simulink model "robusni_of_SMC_regulacija_nelin_sim"  (R2020a)
settings: Solver=ode5  StartTime=0.0  StopTime=tfin  FixedStep=1e-4  RelTol=1e-3
values from neighbouring files (symbols this model uses):
  beta = S_upper_limit*w0/2    (= 0.065530125)    [SMC_regulacija_nelin_sim_matlab.m]    (also in robusni_of_SMC_regulacija_nelin_sim_matlab.m)
  disturb_X = 0.2*Xe    (= 0.97814)    [SMC_regulacija_nelin_sim_matlab.m]    (also in robusni_of_SMC_regulacija_nelin_sim_matlab.m)
  F_lower_limit = 0    [SMC_regulacija_nelin_sim_matlab.m]    (also in robusni_of_SMC_regulacija_nelin_sim_matlab.m)
  F_upper_limit = Fe+1e-3*Fe    (= 3.2121089)    [SMC_regulacija_nelin_sim_matlab.m]    (also in robusni_of_SMC_regulacija_nelin_sim_matlab.m)
  Fi = beta/5/w0    (= 0.02325)    [SMC_regulacija_nelin_sim_matlab.m]    (also in robusni_of_SMC_regulacija_nelin_sim_matlab.m)
  K1 = 0.03    [SMC_regulacija_nelin_sim_matlab.m]    (also in robusni_of_SMC_regulacija_nelin_sim_matlab.m)
  K2 = 0.5    [SMC_regulacija_nelin_sim_matlab.m]    (also in robusni_of_SMC_regulacija_nelin_sim_matlab.m)
  mi_max = 1    [SMC_regulacija_nelin_sim_matlab.m]    (also in robusni_of_SMC_regulacija_nelin_sim_matlab.m)
  S_step = 0    [SMC_regulacija_nelin_sim_matlab.m]    (also in robusni_of_SMC_regulacija_nelin_sim_matlab.m)
  S_time_step1 = 2    [SMC_regulacija_nelin_sim_matlab.m]    (also in robusni_of_SMC_regulacija_nelin_sim_matlab.m = 20)
  S_time_step2 = 40    [SMC_regulacija_nelin_sim_matlab.m]    (also in robusni_of_SMC_regulacija_nelin_sim_matlab.m = 50)
  Se = 0.2187    [SMC_regulacija_nelin_sim_matlab.m]    (also in robusni_of_SMC_regulacija_nelin_sim_matlab.m)
  SF = 10    [SMC_regulacija_nelin_sim_matlab.m]    (also in robusni_of_SMC_regulacija_nelin_sim_matlab.m)
  std_noise = 0    [SMC_regulacija_nelin_sim_matlab.m]    (also in robusni_of_SMC_regulacija_nelin_sim_matlab.m)
  V = 4    [SMC_regulacija_nelin_sim_matlab.m]    (also in robusni_of_SMC_regulacija_nelin_sim_matlab.m)
  x10 = Xe    (= 4.8907)    [SMC_regulacija_nelin_sim_matlab.m]    (also in robusni_of_SMC_regulacija_nelin_sim_matlab.m)
  x20 = Se    (= 0.2187)    [SMC_regulacija_nelin_sim_matlab.m]    (also in robusni_of_SMC_regulacija_nelin_sim_matlab.m)
  Y = 0.5    [SMC_regulacija_nelin_sim_matlab.m]    (also in robusni_of_SMC_regulacija_nelin_sim_matlab.m)
  Y1 = Y - 0.2*Y    (= 0.4)    [robusni_of_SMC_regulacija_nelin_sim_matlab.m]
  Y2 = Y - 0.1*Y    (= 0.45)    [robusni_of_SMC_regulacija_nelin_sim_matlab.m]
  Y3 = Y + 0.1*Y    (= 0.55)    [robusni_of_SMC_regulacija_nelin_sim_matlab.m]
  Y4 = Y + 0.2*Y    (= 0.6)    [robusni_of_SMC_regulacija_nelin_sim_matlab.m]
undefined symbols (not defined in the file or in its folder): magnitude
settings Model: Creator=anaMceranic  LastModifiedBy=anaMceranic
settings DataIOCC: ReturnWorkspaceOutputs=off

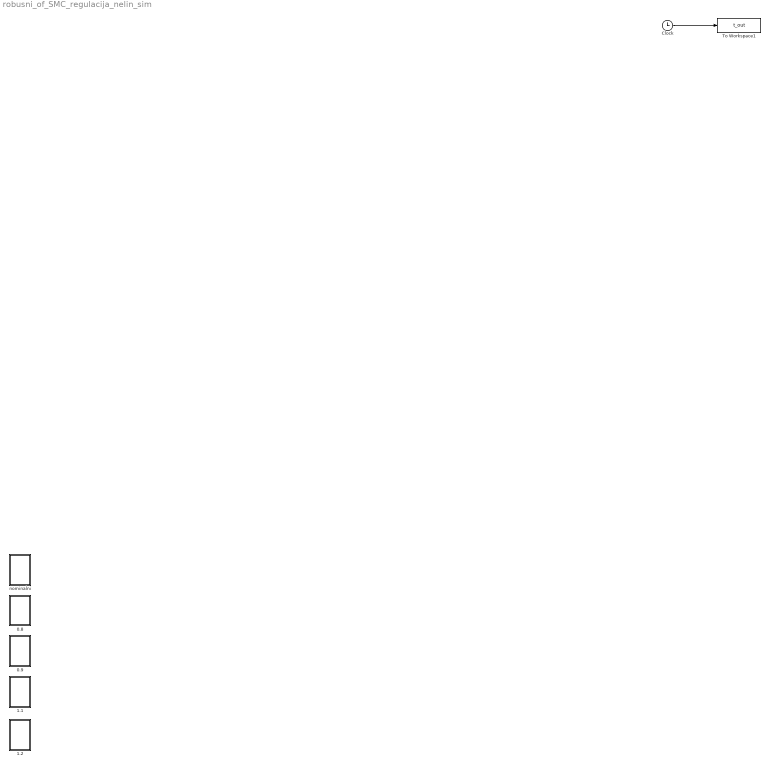
== system robusni_of_SMC_regulacija_nelin_sim ==
  0.8 : Subsystem
  0.9 : Subsystem
  1.1 : Subsystem
  1.2 : Subsystem
  Clock : Clock
  To Workspace1 : ToWorkspace  VariableName=t_out  SampleTime=-1
  nominalni : Subsystem
  wires:
  Clock/1 -> To Workspace1/1

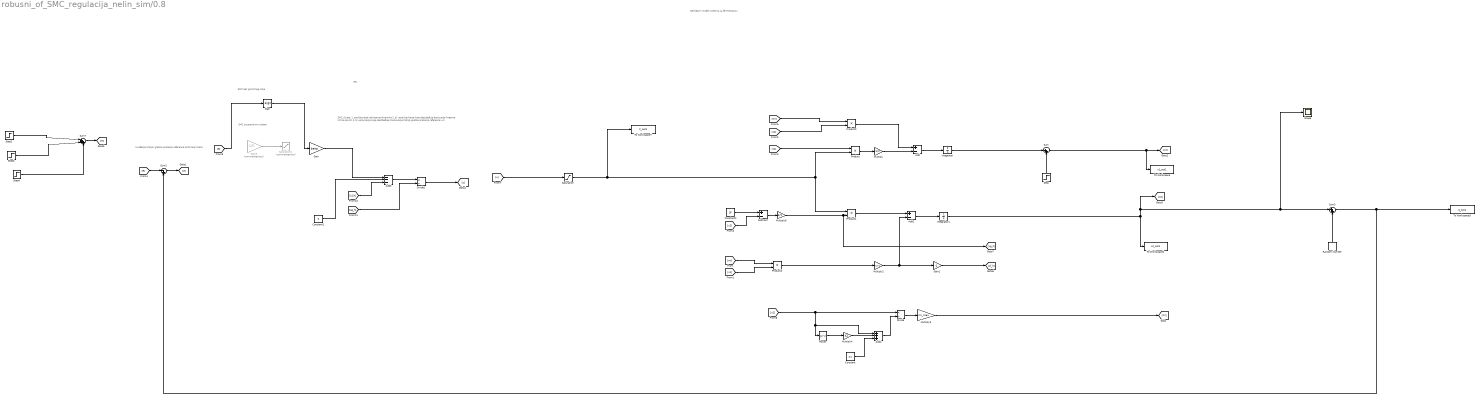
== system robusni_of_SMC_regulacija_nelin_sim/0.8 ==
  note: Nelinearni model sistema za fermentaciju
  note: SMC skupa:
      | 1. poništavanje nelinearne dinamike
      | 2. a) upravljavljanje koje obezbeđuje dostizanje linearne klizne površi
      | 2. b) upravljanje koje obezbeđuje zavšavanje stanja greške praćenja reference u 0
  note: eFL
  note: SMC bez graničnog sloja
  note: SMC sa graničnim slojem
  note: Uvođenje stanja:
      | greška praćenja reference od strane izlaza
  Add : Sum  Inputs=+-
  Add1 : Sum  Inputs=+-
  Add2 : Sum  Inputs=+++
  Add3 : Sum  Inputs=---
  Constant : Constant  Value=K1
  Constant1 : Constant  Value=0
  Constant2 : Constant  Value=SF
  Divide : Product  Inputs=*/
  Divide1 : Product  Inputs=*/
  Gain : Gain  Gain=beta
  Gain1 : Gain  Gain=-1
  Gain3 : Gain  Commented=on  Gain=1/Fi
  Integrator : Integrator  InitialCondition=x10
  Integrator1 : Integrator  InitialCondition=x20
  Multiply : Gain  Gain=1/V
  Multiply2 : Gain  Gain=1/Y1
  Multiply3 : Gain  Gain=mi_max
  Multiply4 : Gain  Gain=K2
  Multiply6 : Gain  Gain=1/V
  Power : Math  Operator=magnitude^2  SaturateOnIntegerOverflow=on
  Product{,1..3} (4 alike) : Product
  Random Number : RandomNumber  Variance=std_noise  SampleTime=0.1
  Saturation : Saturate  UpperLimit=F_upper_limit  LowerLimit=F_lower_limit
  Saturation1 : Saturate  Commented=on
  Scope : Scope
  Sign : Signum
  Step : Step  Time=5  After=disturb_X  SampleTime=0
  Step2 : Step  Time=0  Before=Se  After=Se  SampleTime=0
  Step3 : Step  Time=S_time_step1  After=S_step  SampleTime=0
  Step4 : Step  Time=S_time_step2  After=-S_step  SampleTime=0
  Subtract : Sum  Inputs=+-
  Sum : Sum  Inputs=|++
  Sum2 : Sum  Inputs=|-+
  Sum3 : Sum  Inputs=|++
  Sum7 : Sum  Inputs=|+++
  To Workspace : ToWorkspace  VariableName=x1_out1  SampleTime=-1
  To Workspace2 : ToWorkspace  VariableName=x2_out1  SampleTime=-1
  To Workspace3 : ToWorkspace  VariableName=S_out1  SampleTime=-1
  To Workspace7 : ToWorkspace  VariableName=F_out1  SampleTime=-1
  wires:
  [u] -> Saturation/1
  Random Number/1 -> Sum3/2
  [mi] -> Product3/1
  Product/1 -> Multiply/1
  Add3/1 -> Divide1/1
  Sum2/1 -> [e]
  Divide/1 -> Multiply3/1
  Add/1 -> Integrator/1
  Divide1/1 -> [u]
  Add1/1 -> Integrator1/1
  Product1/1 -> Add1/1
  Integrator/1 -> Sum/1
  Multiply4/1 -> Add2/2
  Constant2/1 -> Subtract/1
  Multiply6/1 -> Product1/2, [Lg_h]
  Constant/1 -> Add2/3
  [x1] -> Product/1
  Step/1 -> Sum/2
  [x2] -> Divide/1, Add2/1, Power/1
  [Lf_h] -> Add3/3
  [x2] -> Subtract/2
  Product2/1 -> Multiply2/1
  Add2/1 -> Divide/2
  Gain3/1 -> Saturation1/1
  Sum/1 -> To Workspace/1, [x1]
  [x1] -> Product3/2
  Sum3/1 -> To Workspace3/1, Sum2/2
  Step4/1 -> Sum7/3
  Integrator1/1 -> To Workspace2/1, [x2], Sum3/1, Scope/1
  Multiply3/1 -> [mi]
  [x1] -> Product2/2
  [Lg_h] -> Divide1/2
  Multiply2/1 -> Add1/2, Gain1/1
  Step3/1 -> Sum7/2
  Gain/1 -> Add3/1
  Product3/1 -> Add/1
  [R] -> Sum2/1
  Subtract/1 -> Multiply6/1
  Multiply/1 -> Add/2
  Saturation/1 -> Product/2, Product1/1, To Workspace7/1
  Gain1/1 -> [Lf_h]
  Sum7/1 -> [R]
  Constant1/1 -> Add3/2
  Step2/1 -> Sum7/1
  [mi] -> Product2/1
  Power/1 -> Multiply4/1
  [e] -> Sign/1
  Sign/1 -> Gain/1

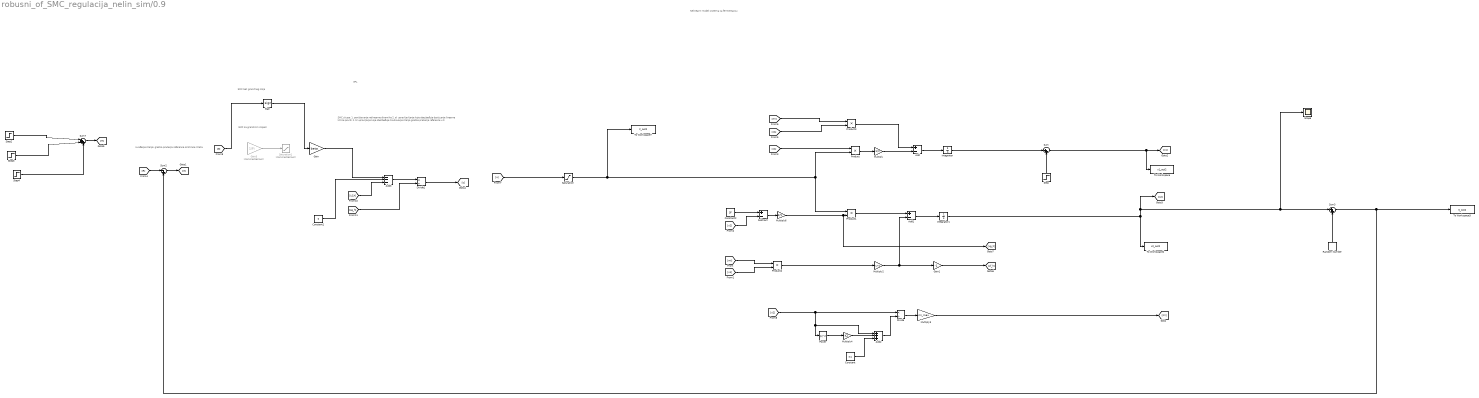
== system robusni_of_SMC_regulacija_nelin_sim/0.9 ==
  note: Uvođenje stanja:
      | greška praćenja reference od strane izlaza
  note: SMC sa graničnim slojem
  note: SMC bez graničnog sloja
  note: eFL
  note: SMC skupa:
      | 1. poništavanje nelinearne dinamike
      | 2. a) upravljavljanje koje obezbeđuje dostizanje linearne klizne površi
      | 2. b) upravljanje koje obezbeđuje zavšavanje stanja greške praćenja reference u 0
  note: Nelinearni model sistema za fermentaciju
  Add : Sum  Inputs=+-
  Add1 : Sum  Inputs=+-
  Add2 : Sum  Inputs=+++
  Add3 : Sum  Inputs=---
  Constant : Constant  Value=K1
  Constant1 : Constant  Value=0
  Constant2 : Constant  Value=SF
  Divide : Product  Inputs=*/
  Divide1 : Product  Inputs=*/
  Gain : Gain  Gain=beta
  Gain1 : Gain  Gain=-1
  Gain3 : Gain  Commented=on  Gain=1/Fi
  Integrator : Integrator  InitialCondition=x10
  Integrator1 : Integrator  InitialCondition=x20
  Multiply : Gain  Gain=1/V
  Multiply2 : Gain  Gain=1/Y2
  Multiply3 : Gain  Gain=mi_max
  Multiply4 : Gain  Gain=K2
  Multiply6 : Gain  Gain=1/V
  Power : Math  Operator=magnitude^2  SaturateOnIntegerOverflow=on
  Product{,1..3} (4 alike) : Product
  Random Number : RandomNumber  Variance=std_noise  SampleTime=0.1
  Saturation : Saturate  UpperLimit=F_upper_limit  LowerLimit=F_lower_limit
  Saturation1 : Saturate  Commented=on
  Scope : Scope
  Sign : Signum
  Step : Step  Time=5  After=disturb_X  SampleTime=0
  Step2 : Step  Time=0  Before=Se  After=Se  SampleTime=0
  Step3 : Step  Time=S_time_step1  After=S_step  SampleTime=0
  Step4 : Step  Time=S_time_step2  After=-S_step  SampleTime=0
  Subtract : Sum  Inputs=+-
  Sum : Sum  Inputs=|++
  Sum2 : Sum  Inputs=|-+
  Sum3 : Sum  Inputs=|++
  Sum7 : Sum  Inputs=|+++
  To Workspace : ToWorkspace  VariableName=x1_out2  SampleTime=-1
  To Workspace2 : ToWorkspace  VariableName=x2_out2  SampleTime=-1
  To Workspace3 : ToWorkspace  VariableName=S_out2  SampleTime=-1
  To Workspace7 : ToWorkspace  VariableName=F_out2  SampleTime=-1
  wires:
  Power/1 -> Multiply4/1
  [mi] -> Product2/1
  Step2/1 -> Sum7/1
  Constant1/1 -> Add3/2
  Sum7/1 -> [R]
  Gain1/1 -> [Lf_h]
  Saturation/1 -> To Workspace7/1, Product1/1, Product/2
  Multiply/1 -> Add/2
  Subtract/1 -> Multiply6/1
  [R] -> Sum2/1
  Product3/1 -> Add/1
  Gain/1 -> Add3/1
  Step3/1 -> Sum7/2
  Multiply2/1 -> Gain1/1, Add1/2
  [Lg_h] -> Divide1/2
  [x1] -> Product2/2
  Multiply3/1 -> [mi]
  Integrator1/1 -> Scope/1, Sum3/1, [x2], To Workspace2/1
  Step4/1 -> Sum7/3
  Sum3/1 -> Sum2/2, To Workspace3/1
  [x1] -> Product3/2
  Sum/1 -> [x1], To Workspace/1
  Gain3/1 -> Saturation1/1
  Add2/1 -> Divide/2
  Product2/1 -> Multiply2/1
  [x2] -> Subtract/2
  [Lf_h] -> Add3/3
  [x2] -> Power/1, Add2/1, Divide/1
  Step/1 -> Sum/2
  [x1] -> Product/1
  Constant/1 -> Add2/3
  Multiply6/1 -> [Lg_h], Product1/2
  Constant2/1 -> Subtract/1
  Multiply4/1 -> Add2/2
  Integrator/1 -> Sum/1
  Product1/1 -> Add1/1
  Add1/1 -> Integrator1/1
  Divide1/1 -> [u]
  Add/1 -> Integrator/1
  Divide/1 -> Multiply3/1
  Sum2/1 -> [e]
  Add3/1 -> Divide1/1
  Product/1 -> Multiply/1
  [mi] -> Product3/1
  Random Number/1 -> Sum3/2
  [u] -> Saturation/1
  [e] -> Sign/1
  Sign/1 -> Gain/1

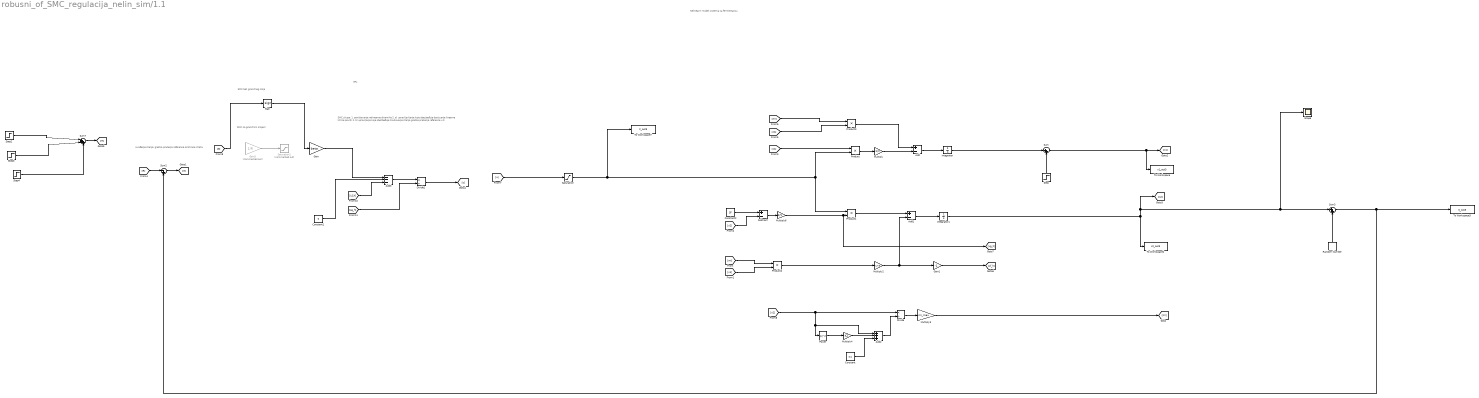
== system robusni_of_SMC_regulacija_nelin_sim/1.1 ==
  note: Nelinearni model sistema za fermentaciju
  note: SMC skupa:
      | 1. poništavanje nelinearne dinamike
      | 2. a) upravljavljanje koje obezbeđuje dostizanje linearne klizne površi
      | 2. b) upravljanje koje obezbeđuje zavšavanje stanja greške praćenja reference u 0
  note: eFL
  note: SMC bez graničnog sloja
  note: SMC sa graničnim slojem
  note: Uvođenje stanja:
      | greška praćenja reference od strane izlaza
  Add : Sum  Inputs=+-
  Add1 : Sum  Inputs=+-
  Add2 : Sum  Inputs=+++
  Add3 : Sum  Inputs=---
  Constant : Constant  Value=K1
  Constant1 : Constant  Value=0
  Constant2 : Constant  Value=SF
  Divide : Product  Inputs=*/
  Divide1 : Product  Inputs=*/
  Gain : Gain  Gain=beta
  Gain1 : Gain  Gain=-1
  Gain3 : Gain  Commented=on  Gain=1/Fi
  Integrator : Integrator  InitialCondition=x10
  Integrator1 : Integrator  InitialCondition=x20
  Multiply : Gain  Gain=1/V
  Multiply2 : Gain  Gain=1/Y3
  Multiply3 : Gain  Gain=mi_max
  Multiply4 : Gain  Gain=K2
  Multiply6 : Gain  Gain=1/V
  Power : Math  Operator=magnitude^2  SaturateOnIntegerOverflow=on
  Product{,1..3} (4 alike) : Product
  Random Number : RandomNumber  Variance=std_noise  SampleTime=0.1
  Saturation : Saturate  UpperLimit=F_upper_limit  LowerLimit=F_lower_limit
  Saturation1 : Saturate  Commented=on
  Scope : Scope
  Sign : Signum
  Step : Step  Time=5  After=disturb_X  SampleTime=0
  Step2 : Step  Time=0  Before=Se  After=Se  SampleTime=0
  Step3 : Step  Time=S_time_step1  After=S_step  SampleTime=0
  Step4 : Step  Time=S_time_step2  After=-S_step  SampleTime=0
  Subtract : Sum  Inputs=+-
  Sum : Sum  Inputs=|++
  Sum2 : Sum  Inputs=|-+
  Sum3 : Sum  Inputs=|++
  Sum7 : Sum  Inputs=|+++
  To Workspace : ToWorkspace  VariableName=x1_out3  SampleTime=-1
  To Workspace2 : ToWorkspace  VariableName=x2_out3  SampleTime=-1
  To Workspace3 : ToWorkspace  VariableName=S_out3  SampleTime=-1
  To Workspace7 : ToWorkspace  VariableName=F_out3  SampleTime=-1
  wires:
  [u] -> Saturation/1
  Random Number/1 -> Sum3/2
  [mi] -> Product3/1
  Product/1 -> Multiply/1
  Add3/1 -> Divide1/1
  Sum2/1 -> [e]
  Divide/1 -> Multiply3/1
  Add/1 -> Integrator/1
  Divide1/1 -> [u]
  Add1/1 -> Integrator1/1
  Product1/1 -> Add1/1
  Integrator/1 -> Sum/1
  Multiply4/1 -> Add2/2
  Constant2/1 -> Subtract/1
  Multiply6/1 -> Product1/2, [Lg_h]
  Constant/1 -> Add2/3
  [x1] -> Product/1
  Step/1 -> Sum/2
  [x2] -> Divide/1, Add2/1, Power/1
  [Lf_h] -> Add3/3
  [x2] -> Subtract/2
  Product2/1 -> Multiply2/1
  Add2/1 -> Divide/2
  Gain3/1 -> Saturation1/1
  Sum/1 -> To Workspace/1, [x1]
  [x1] -> Product3/2
  Sum3/1 -> To Workspace3/1, Sum2/2
  Step4/1 -> Sum7/3
  Integrator1/1 -> To Workspace2/1, [x2], Sum3/1, Scope/1
  Multiply3/1 -> [mi]
  [x1] -> Product2/2
  [Lg_h] -> Divide1/2
  Multiply2/1 -> Add1/2, Gain1/1
  Step3/1 -> Sum7/2
  Gain/1 -> Add3/1
  Product3/1 -> Add/1
  [R] -> Sum2/1
  Subtract/1 -> Multiply6/1
  Multiply/1 -> Add/2
  Saturation/1 -> Product/2, Product1/1, To Workspace7/1
  Gain1/1 -> [Lf_h]
  Sum7/1 -> [R]
  Constant1/1 -> Add3/2
  Step2/1 -> Sum7/1
  [mi] -> Product2/1
  Power/1 -> Multiply4/1
  [e] -> Sign/1
  Sign/1 -> Gain/1

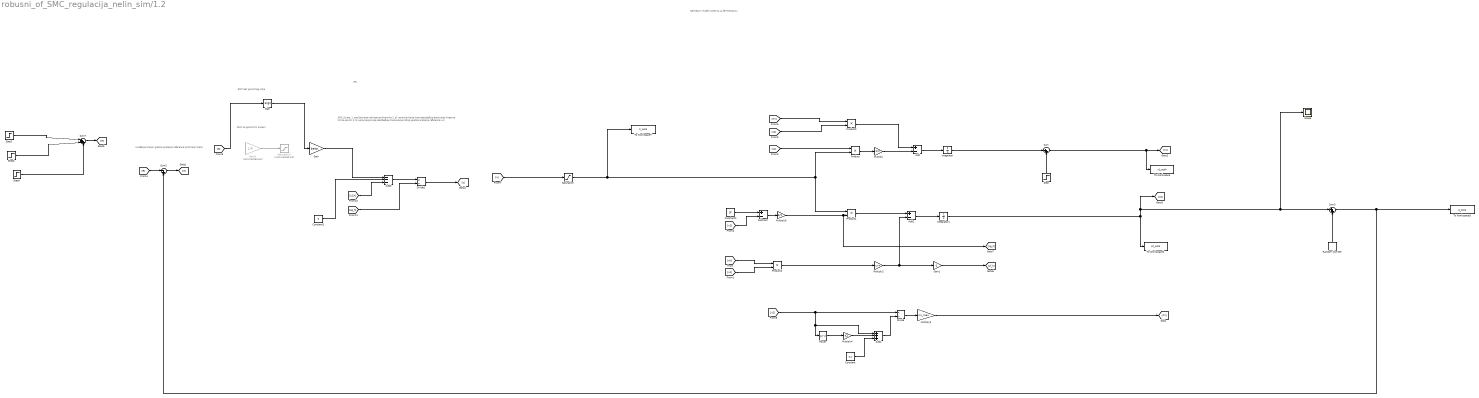
== system robusni_of_SMC_regulacija_nelin_sim/1.2 ==
  note: Uvođenje stanja:
      | greška praćenja reference od strane izlaza
  note: SMC sa graničnim slojem
  note: SMC bez graničnog sloja
  note: eFL
  note: SMC skupa:
      | 1. poništavanje nelinearne dinamike
      | 2. a) upravljavljanje koje obezbeđuje dostizanje linearne klizne površi
      | 2. b) upravljanje koje obezbeđuje zavšavanje stanja greške praćenja reference u 0
  note: Nelinearni model sistema za fermentaciju
  Add : Sum  Inputs=+-
  Add1 : Sum  Inputs=+-
  Add2 : Sum  Inputs=+++
  Add3 : Sum  Inputs=---
  Constant : Constant  Value=K1
  Constant1 : Constant  Value=0
  Constant2 : Constant  Value=SF
  Divide : Product  Inputs=*/
  Divide1 : Product  Inputs=*/
  Gain : Gain  Gain=beta
  Gain1 : Gain  Gain=-1
  Gain3 : Gain  Commented=on  Gain=1/Fi
  Integrator : Integrator  InitialCondition=x10
  Integrator1 : Integrator  InitialCondition=x20
  Multiply : Gain  Gain=1/V
  Multiply2 : Gain  Gain=1/Y4
  Multiply3 : Gain  Gain=mi_max
  Multiply4 : Gain  Gain=K2
  Multiply6 : Gain  Gain=1/V
  Power : Math  Operator=magnitude^2  SaturateOnIntegerOverflow=on
  Product{,1..3} (4 alike) : Product
  Random Number : RandomNumber  Variance=std_noise  SampleTime=0.1
  Saturation : Saturate  UpperLimit=F_upper_limit  LowerLimit=F_lower_limit
  Saturation1 : Saturate  Commented=on
  Scope : Scope
  Sign : Signum
  Step : Step  Time=5  After=disturb_X  SampleTime=0
  Step2 : Step  Time=0  Before=Se  After=Se  SampleTime=0
  Step3 : Step  Time=S_time_step1  After=S_step  SampleTime=0
  Step4 : Step  Time=S_time_step2  After=-S_step  SampleTime=0
  Subtract : Sum  Inputs=+-
  Sum : Sum  Inputs=|++
  Sum2 : Sum  Inputs=|-+
  Sum3 : Sum  Inputs=|++
  Sum7 : Sum  Inputs=|+++
  To Workspace : ToWorkspace  VariableName=x1_out4  SampleTime=-1
  To Workspace2 : ToWorkspace  VariableName=x2_out4  SampleTime=-1
  To Workspace3 : ToWorkspace  VariableName=S_out4  SampleTime=-1
  To Workspace7 : ToWorkspace  VariableName=F_out4  SampleTime=-1
  wires:
  Power/1 -> Multiply4/1
  [mi] -> Product2/1
  Step2/1 -> Sum7/1
  Constant1/1 -> Add3/2
  Sum7/1 -> [R]
  Gain1/1 -> [Lf_h]
  Saturation/1 -> To Workspace7/1, Product1/1, Product/2
  Multiply/1 -> Add/2
  Subtract/1 -> Multiply6/1
  [R] -> Sum2/1
  Product3/1 -> Add/1
  Gain/1 -> Add3/1
  Step3/1 -> Sum7/2
  Multiply2/1 -> Gain1/1, Add1/2
  [Lg_h] -> Divide1/2
  [x1] -> Product2/2
  Multiply3/1 -> [mi]
  Integrator1/1 -> Scope/1, Sum3/1, [x2], To Workspace2/1
  Step4/1 -> Sum7/3
  Sum3/1 -> Sum2/2, To Workspace3/1
  [x1] -> Product3/2
  Sum/1 -> [x1], To Workspace/1
  Gain3/1 -> Saturation1/1
  Add2/1 -> Divide/2
  Product2/1 -> Multiply2/1
  [x2] -> Subtract/2
  [Lf_h] -> Add3/3
  [x2] -> Power/1, Add2/1, Divide/1
  Step/1 -> Sum/2
  [x1] -> Product/1
  Constant/1 -> Add2/3
  Multiply6/1 -> [Lg_h], Product1/2
  Constant2/1 -> Subtract/1
  Multiply4/1 -> Add2/2
  Integrator/1 -> Sum/1
  Product1/1 -> Add1/1
  Add1/1 -> Integrator1/1
  Divide1/1 -> [u]
  Add/1 -> Integrator/1
  Divide/1 -> Multiply3/1
  Sum2/1 -> [e]
  Add3/1 -> Divide1/1
  Product/1 -> Multiply/1
  [mi] -> Product3/1
  Random Number/1 -> Sum3/2
  [u] -> Saturation/1
  [e] -> Sign/1
  Sign/1 -> Gain/1

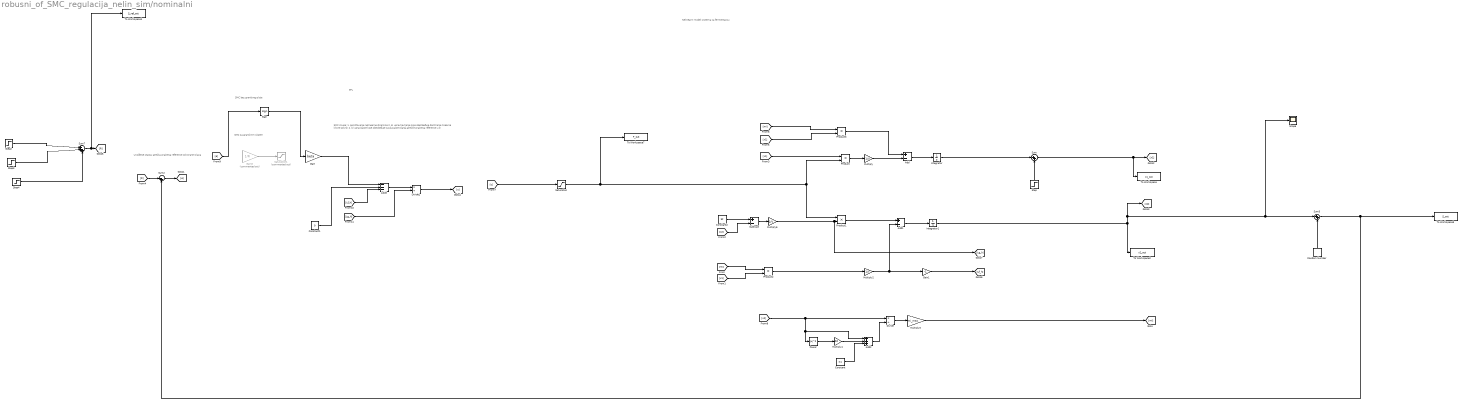
== system robusni_of_SMC_regulacija_nelin_sim/nominalni ==
  note: Uvođenje stanja:
      | greška praćenja reference od strane izlaza
  note: SMC sa graničnim slojem
  note: SMC bez graničnog sloja
  note: eFL
  note: SMC skupa:
      | 1. poništavanje nelinearne dinamike
      | 2. a) upravljavljanje koje obezbeđuje dostizanje linearne klizne površi
      | 2. b) upravljanje koje obezbeđuje zavšavanje stanja greške praćenja reference u 0
  note: Nelinearni model sistema za fermentaciju
  Add : Sum  Inputs=+-
  Add1 : Sum  Inputs=+-
  Add2 : Sum  Inputs=+++
  Add3 : Sum  Inputs=---
  Constant : Constant  Value=K1
  Constant1 : Constant  Value=0
  Constant2 : Constant  Value=SF
  Divide : Product  Inputs=*/
  Divide1 : Product  Inputs=*/
  Gain : Gain  Gain=beta
  Gain1 : Gain  Gain=-1
  Gain3 : Gain  Commented=on  Gain=1/Fi
  Integrator : Integrator  InitialCondition=x10
  Integrator1 : Integrator  InitialCondition=x20
  Multiply : Gain  Gain=1/V
  Multiply2 : Gain  Gain=1/Y
  Multiply3 : Gain  Gain=mi_max
  Multiply4 : Gain  Gain=K2
  Multiply6 : Gain  Gain=1/V
  Power : Math  Operator=magnitude^2  SaturateOnIntegerOverflow=on
  Product{,1..3} (4 alike) : Product
  Random Number : RandomNumber  Variance=std_noise  SampleTime=0.1
  Saturation : Saturate  UpperLimit=F_upper_limit  LowerLimit=F_lower_limit
  Saturation1 : Saturate  Commented=on
  Scope : Scope
  Sign : Signum
  Step : Step  Time=5  After=disturb_X  SampleTime=0
  Step2 : Step  Time=0  Before=Se  After=Se  SampleTime=0
  Step3 : Step  Time=S_time_step1  After=S_step  SampleTime=0
  Step4 : Step  Time=S_time_step2  After=-S_step  SampleTime=0
  Subtract : Sum  Inputs=+-
  Sum : Sum  Inputs=|++
  Sum2 : Sum  Inputs=|-+
  Sum3 : Sum  Inputs=|++
  Sum7 : Sum  Inputs=|+++
  To Workspace : ToWorkspace  VariableName=x1_out  SampleTime=-1
  To Workspace1 : ToWorkspace  VariableName=S_ref_out  SampleTime=-1
  To Workspace2 : ToWorkspace  VariableName=x2_out  SampleTime=-1
  To Workspace3 : ToWorkspace  VariableName=S_out  SampleTime=-1
  To Workspace7 : ToWorkspace  VariableName=F_out  SampleTime=-1
  wires:
  Power/1 -> Multiply4/1
  [mi] -> Product2/1
  Step2/1 -> Sum7/1
  Constant1/1 -> Add3/2
  Sum7/1 -> To Workspace1/1, [R]
  Gain1/1 -> [Lf_h]
  Saturation/1 -> To Workspace7/1, Product1/1, Product/2
  Multiply/1 -> Add/2
  Subtract/1 -> Multiply6/1
  [R] -> Sum2/1
  Product3/1 -> Add/1
  Gain/1 -> Add3/1
  Step3/1 -> Sum7/2
  Multiply2/1 -> Gain1/1, Add1/2
  [Lg_h] -> Divide1/2
  [x1] -> Product2/2
  Multiply3/1 -> [mi]
  Integrator1/1 -> Scope/1, Sum3/1, [x2], To Workspace2/1
  Step4/1 -> Sum7/3
  Sum3/1 -> Sum2/2, To Workspace3/1
  [x1] -> Product3/2
  Sum/1 -> [x1], To Workspace/1
  Gain3/1 -> Saturation1/1
  Add2/1 -> Divide/2
  Product2/1 -> Multiply2/1
  [x2] -> Subtract/2
  [Lf_h] -> Add3/3
  [x2] -> Power/1, Add2/1, Divide/1
  Step/1 -> Sum/2
  [x1] -> Product/1
  Constant/1 -> Add2/3
  Multiply6/1 -> [Lg_h], Product1/2
  Constant2/1 -> Subtract/1
  Multiply4/1 -> Add2/2
  Integrator/1 -> Sum/1
  Product1/1 -> Add1/1
  Add1/1 -> Integrator1/1
  Divide1/1 -> [u]
  Add/1 -> Integrator/1
  Divide/1 -> Multiply3/1
  Sum2/1 -> [e]
  Add3/1 -> Divide1/1
  Product/1 -> Multiply/1
  [mi] -> Product3/1
  Random Number/1 -> Sum3/2
  [u] -> Saturation/1
  [e] -> Sign/1
  Sign/1 -> Gain/1
